simulink model "BDOT"  (R2021a)
settings: Solver=ode4  StartTime=0.0  StopTime=duration  FixedStep=dt  RelTol=1e-3
InitFcn:
  | init_param
values from neighbouring files (symbols this model uses):
  h0 = zeros(3,1)    [init_param.m]
  init_pv_eci = [-5877328.551 3688970.336 11369.332  550.193937 853.430111 7510.746227]    [init_param.m]
  jd0 = DateTime2JD(epoch)    [init_param.m]
  L0 = Ib*w0    [init_param.m]
  mtq_thd = 0.48    [init_param.m]
  Qi2b0 = [1 0 0 0]'    [init_param.m]
  r2d = 1/deg2rad    (= 57.2957795131)    [init_param.m]
settings Model: Creator=kozak  LastModifiedBy=kozak
settings DataIOCC: SaveOutput=off  SignalLogging=off  DSMLogging=off  SaveTime=off  ReturnWorkspaceOutputs=off

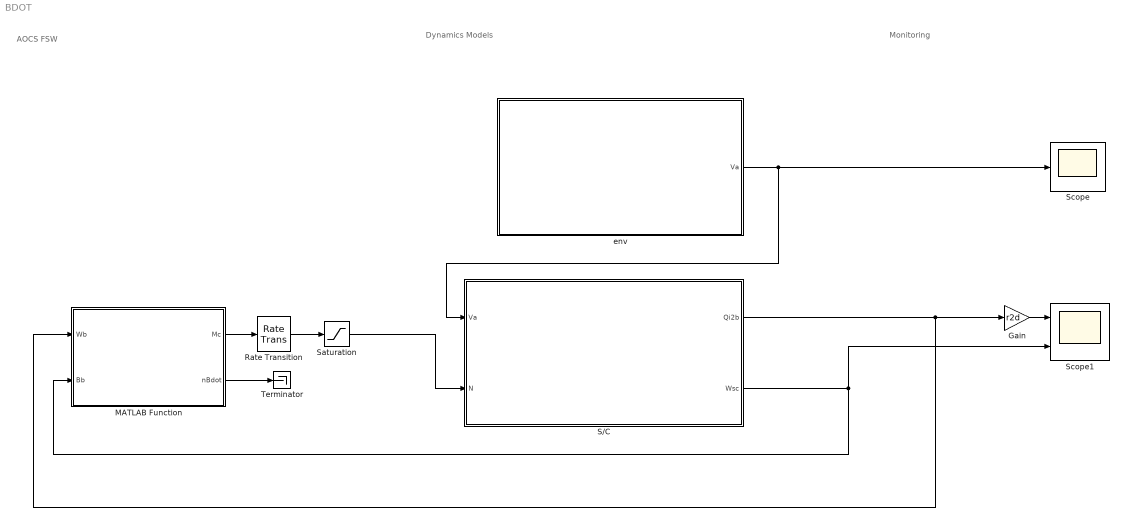
== system BDOT ==
  note: Monitoring
  note: Dynamics Models
  note: AOCS FSW
  Gain : Gain  Gain=r2d
  MATLAB Function : MATLAB Function  TreatAsAtomicUnit=on
  Rate Transition : RateTransition  OutPortSampleTime=bdot_cycle
  S/C : Subsystem
  Saturation : Saturate  UpperLimit=mtq_thd
  Scope : Scope
  Scope1 : Scope  NumInputPorts=2
  Terminator : Terminator
  env : Subsystem
  wires:
  env/1(Va) -> S/C/1(Va), Scope/1
  S/C/2(Wsc) -> MATLAB Function/2(Bb), Scope1/2
  MATLAB Function/1(Mc) -> Rate Transition/1
  Rate Transition/1 -> Saturation/1
  MATLAB Function/2(nBdot) -> Terminator/1
  Saturation/1 -> S/C/2(N)
  Gain/1 -> Scope1/1
  S/C/1(Qi2b) -> Gain/1, MATLAB Function/1(Wb)

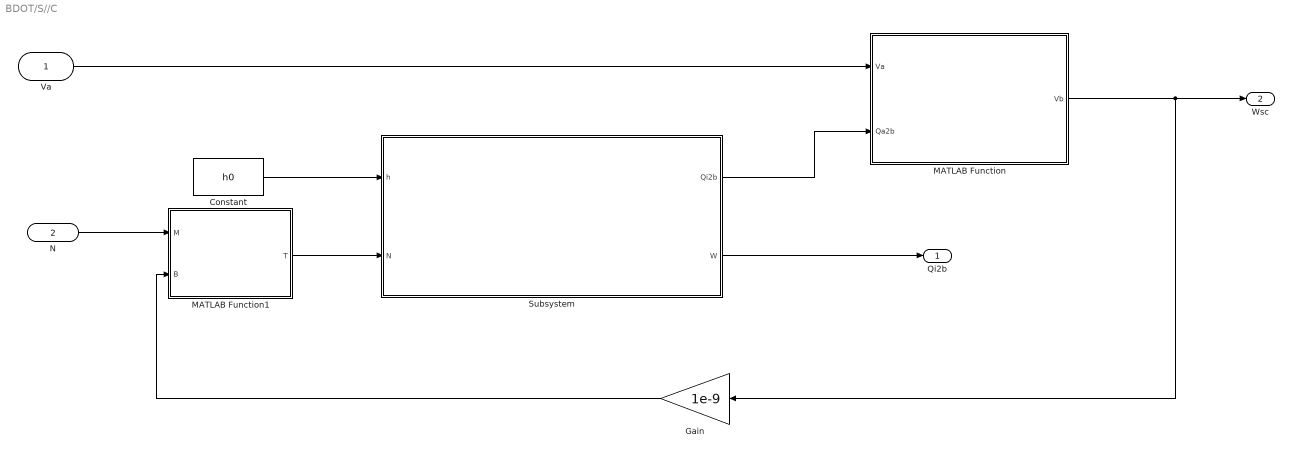
== system BDOT/S//C ==
  Va : Inport
  N : Inport  Port=2
  Constant : Constant  Value=h0
  Gain : Gain  Gain=1e-9
  MATLAB Function : MATLAB Function  TreatAsAtomicUnit=on
  MATLAB Function1 : MATLAB Function  TreatAsAtomicUnit=on
  Subsystem : Subsystem
  Qi2b : Outport
  Wsc : Outport  Port=2
  wires:
  Va/1 -> MATLAB Function/1(Va)
  Subsystem/1(Qi2b) -> MATLAB Function/2(Qa2b)
  MATLAB Function/1(Vb) -> Wsc/1, Gain/1
  N/1 -> MATLAB Function1/1(M)
  Gain/1 -> MATLAB Function1/2(B)
  MATLAB Function1/1(T) -> Subsystem/2(N)
  Constant/1 -> Subsystem/1(h)
  Subsystem/2(W) -> Qi2b/1

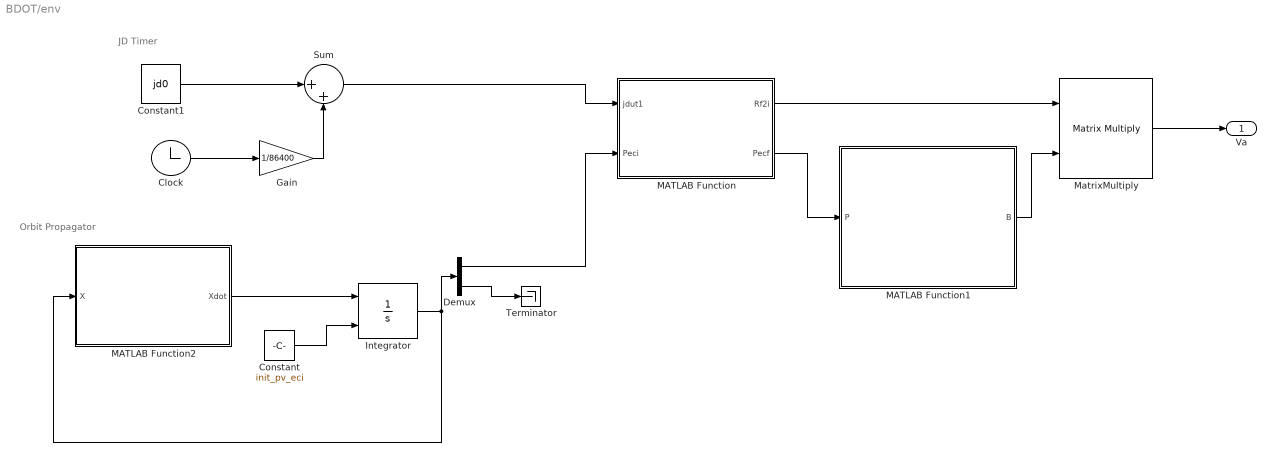
== system BDOT/env ==
  note: Orbit Propagator
  note: JD Timer
  Clock : Clock
  Constant : Constant  Value=init_pv_eci
  Constant1 : Constant  Value=jd0
  Demux : Demux  Outputs=2
  Gain : Gain  Gain=1/86400
  Integrator : Integrator  InitialConditionSource=external
  MATLAB Function : MATLAB Function  TreatAsAtomicUnit=on
  MATLAB Function1 : MATLAB Function  TreatAsAtomicUnit=on
  MATLAB Function2 : MATLAB Function  TreatAsAtomicUnit=on
  MatrixMultiply : Product  Multiplication=Matrix(*)
  Sum : Sum  Inputs=|++
  Terminator : Terminator
  Va : Outport
  wires:
  Demux/2 -> Terminator/1
  Integrator/1 -> MATLAB Function2/1(X), Demux/1
  Constant/1 -> Integrator/2
  Sum/1 -> MATLAB Function/1(jdut1)
  Constant1/1 -> Sum/1
  MATLAB Function/2(Pecf) -> MATLAB Function1/1(P)
  Demux/1 -> MATLAB Function/2(Peci)
  Gain/1 -> Sum/2
  Clock/1 -> Gain/1
  MatrixMultiply/1 -> Va/1
  MATLAB Function1/1(B) -> MatrixMultiply/2
  MATLAB Function2/1(Xdot) -> Integrator/1
  MATLAB Function/1(Rf2i) -> MatrixMultiply/1

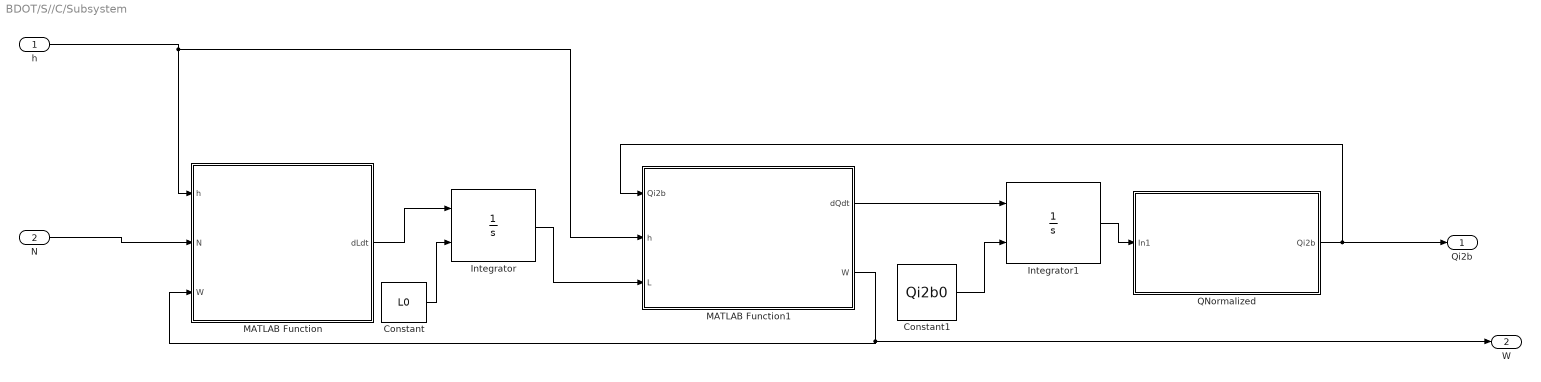
== system BDOT/S//C/Subsystem ==
  h : Inport
  N : Inport  Port=2
  Constant : Constant  Value=L0
  Constant1 : Constant  Value=Qi2b0
  Integrator : Integrator  InitialConditionSource=external
  Integrator1 : Integrator  InitialConditionSource=external
  MATLAB Function : MATLAB Function
  MATLAB Function1 : MATLAB Function  TreatAsAtomicUnit=on
  QNormalized : Subsystem
  Qi2b : Outport
  W : Outport  Port=2
  wires:
  MATLAB Function1/2(W) -> W/1, MATLAB Function/3(W)
  Integrator/1 -> MATLAB Function1/3(L)
  QNormalized/1(Qi2b) -> Qi2b/1, MATLAB Function1/1(Qi2b)
  MATLAB Function1/1(dQdt) -> Integrator1/1
  Constant/1 -> Integrator/2
  Integrator1/1 -> QNormalized/1(In1)
  MATLAB Function/1(dLdt) -> Integrator/1
  h/1 -> MATLAB Function/1(h), MATLAB Function1/2(h)
  Constant1/1 -> Integrator1/2
  N/1 -> MATLAB Function/2(N)

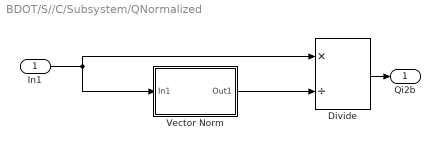
== system BDOT/S//C/Subsystem/QNormalized ==
  In1 : Inport
  Divide : Product  Inputs=*/
  Vector Norm : Subsystem
  Qi2b : Outport
  wires:
  In1/1 -> Divide/1, Vector Norm/1(In1)
  Divide/1 -> Qi2b/1
  Vector Norm/1(Out1) -> Divide/2

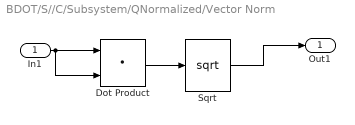
== system BDOT/S//C/Subsystem/QNormalized/Vector Norm ==
  In1 : Inport
  Dot Product : DotProduct  InputSameDT=on  OutDataTypeStr=Inherit: Inherit via internal rule
  Sqrt : Sqrt  SaturateOnIntegerOverflow=on
  Out1 : Outport
  wires:
  Dot Product/1 -> Sqrt/1
  In1/1 -> Dot Product/2, Dot Product/1
  Sqrt/1 -> Out1/1

== matlab function BDOT/env/MATLAB Function1 ==
  data: P input; B output; mpm parameter
function B = MagneticDipole(P, mpm)
re = 6371e3; %m
mu0 = 4*pi*1e-7; %N/A^2
m =((4*pi*re^3/mu0).*[mpm.g11 mpm.h11 mpm.g10])';
k0 = mu0*m/(4*pi);
Pnorm = norm(P);
R = P/Pnorm;
y = (3*(R'*k0)*R-k0)/Pnorm^3; % T
B = y*1e9; %nT

== matlab function BDOT/env/MATLAB Function ==
  data: jdut1 input; Rf2i output; Peci input; Pecf output
%% ECI to ECEF Transformation
function [Rf2i, Pecf] = ECI2ECF(jdut1, Peci)
Ri2f = R3(JD2GMST(jdut1));
Pecf = Ri2f*Peci; %in m
Rf2i = Ri2f';

== matlab function BDOT/env/MATLAB Function2 ==
  data: X input; Xdot output; mu_e parameter
function Xdot = TwoBodyRHS(X, mu_e)
r = X(1:3);
v = X(4:6);
Xdot=[v; -(mu_e*r/norm(r)^3)];

== matlab function BDOT/S//C/Subsystem/MATLAB Function ==
  data: h input; dLdt output; N input; W input; Ib parameter
%% Euler Equation
function dLdt= EulerEquation(h,N,W,Ib)
L = Ib*W + h;
dLdt = N-cross((Ib\(L-h)),L);

== matlab function BDOT/S//C/Subsystem/MATLAB Function1 ==
  data: Qi2b input; dQdt output; h input; L input; W output; Ib parameter
%% Quaternion Kinematic Equation
function [dQdt, W] = QuatKinematic(Qi2b,h,L, Ib)
W =Ib\(L-h);
dQdt = 0.5 * (QMul(Qi2b,[0;W]));

== matlab function BDOT/S//C/MATLAB Function ==
  data: Va input; Vb output; Qa2b input
%% convert a vector in A frame to that in B frame by the quaternion operator
function Vb = EciToBody(Va,Qa2b)
Qb2a = QInv(Qa2b);
qout = QMul(QMul(Qb2a, [0;Va]), Qa2b);
Vb = [qout(2) qout(3) qout(4)]';

== matlab function BDOT/MATLAB Function ==
  data: Wb input; Mc output; Bb input; nBdot output; k parameter
%% Bdot Control 
function [Mc,nBdot] = Bdot(Wb, Bb, k)
Bdot = -cross(Wb,Bb);
nBdot = norm(Bdot);
% divided-by-zero check
if abs(nBdot-eps)> 1e-5
bdot = Bdot/nBdot;
else
bdot = zeros(3,1);
end
Mc = -(k*norm(Wb))*bdot;

== matlab function BDOT/S//C/MATLAB Function1 ==
  data: M input; T output; B input
function T = MXB(M,B)
T = cross(M,B);
